simulink model "Controller1_PD"  (R2021b)
settings: Solver=ode45  StartTime=0.0  StopTime=15  RelTol=1e-3
libraries: simulink_extras x1
settings Model: Creator=david  LastModifiedBy=david

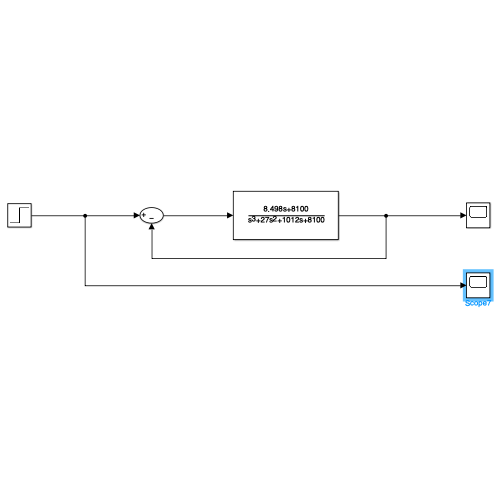
[thumbnail: Simulink's stored preview of the top-level diagram]
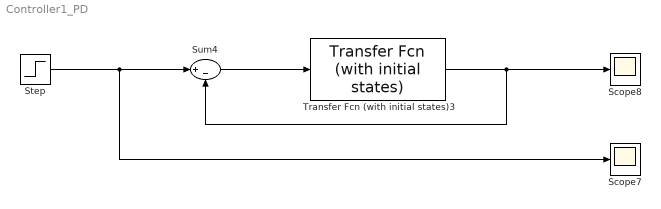
== system Controller1_PD ==
  Scope7 : Scope
  Scope8 : Scope
  Step : Step  SampleTime=0
  Sum4 : Sum  Inputs=|+-
  Transfer Fcn (with initial states)3 : simulink_extras/Additional Linear/Transfer Fcn (with initial states)  N=[8.498 8100]  D=[1 27 1012 8100]  X0=0
  wires:
  Transfer Fcn (with initial states)3/1 -> Sum4/2, Scope8/1
  Sum4/1 -> Transfer Fcn (with initial states)3/1
  Step/1 -> Scope7/1, Sum4/1
